simulink model "PubIfDecisionVSM_LngHMI"  (R2020b)
settings: Solver=FixedStepAuto  StartTime=0.0  StopTime=Inf  RelTol=1e-3
PostLoadFcn:
  | if any(exist('dsrtsu_mdlpostloadfcn', 'file') ~= 0), dsrtsu_mdlpostloadfcn('Execute', bdroot); end
InitFcn:
  | , if any(exist('dsmpb_private', 'file') ~= 0), dsmpb_private('dsmpb_mdlclblib', 'Init', bdroot); end,
PreSaveFcn:
  | , if any(exist('dsmpb_private', 'file') ~= 0), dsmpb_private('dsmpb_mdlclblib', 'PreSave', bdroot); end,
CloseFcn:
  | , if any(exist('dsmpb_private', 'file') ~= 0), dsmpb_private('dsmpb_mdlclblib', 'Close', bdroot); end,
settings Model: DataDictionary=HWA_DDs.sldd  RTICANMMDATA=struct('GeneralSetupData',struct('modelroot','F:\ADAS_Store\ADAS_Store\Adas\VSM\Long_HMI','generalsettings',struct('filesettings',struct('destfolder',struct('Name','RTICANMM_FILES','Check',1),'buildfolder',struct('Name','.','Check',1),'AbsDestfolder',struct('Name','F:\ADAS_Store\ADAS_Store\Adas\VSM\Long_HMI\RTICANMM_FILES'),'AbsBuildfolder',struct('Name','F:\ADAS_Store\ADAS_Store\Adas\VSM\Long_HMI'))),'options',struct('addpaths',1,'rmpaths',1,'addtrcexclusion',false,'cannavigator',struct('checkmonitoring',0),'show_usrtrc',0,'use_usrtrc',0),'advanced',struct('options',ones(1,100)),'MPSetup',{{}},'RTI',struct('Type','DSRT','Ver','4.2','Date','02-Nov-2019'),'modelname','PubIfDecisionVSM_LngHMI','block','PubIfDecisionVSM_LngHMI'))  DSRTSU_INTERNAL_RTIFPGA=150  Creator=GW00180895  LastModifiedBy=GW00199575
settings OptimizationCC: BlockReduction=off  ConditionallyExecuteInputs=off  OptimizeBlockIOStorage=off  BufferReuse=off  GlobalBufferReuse=off  ExpressionFolding=off  LocalBlockOutputs=off  OptimizeDataStoreBuffers=off  BusAssignmentInplaceUpdate=off
settings DebuggingCC: TasksWithSamePriorityMsg=none
settings HardwareCC: ProdBitPerPointer=32  ProdBitPerSizeT=32  ProdBitPerPtrDiffT=32  ProdLargestAtomicInteger=Integer  ProdWordSize=32  ProdHWDeviceType=Custom Processor->Custom
settings ModelReferenceCC: UpdateModelReferenceTargets=IfOutOfDate  EnableParallelModelReferenceBuilds=on  ModelReferenceNumInstancesAllowed=Single
settings SFSimCC: MATLABDynamicMemAlloc=off
settings RTWCC: Description=dSPACE Run-Time Target (for VEOS on Windows and ConfigurationDesk)  SystemTargetFile=dsrt.tlc  GenCodeOnly=on  MakeCommand=make_dsrt  TemplateMakefile=dsrt_default_tmf  RTWVerbose=off
settings CodeAppCC: MaxIdLength=128
settings STFCustomTargetCC: TargetLangStandard=C99 (ISO)  ParMdlRefBuildCompliant=on  ConcurrentExecutionCompliant=off  CPPClassGenCompliant=off  GRTInterface=off  SystemTargetFile=dsrt.tlc
settings GRTTargetCC: CompOptLevelCompliant=off  ConcurrentExecutionCompliant=off  CombineOutputUpdateFcns=off  MatFileLogging=off  CPPClassGenCompliant=off  UseToolchainInfoCompliant=off

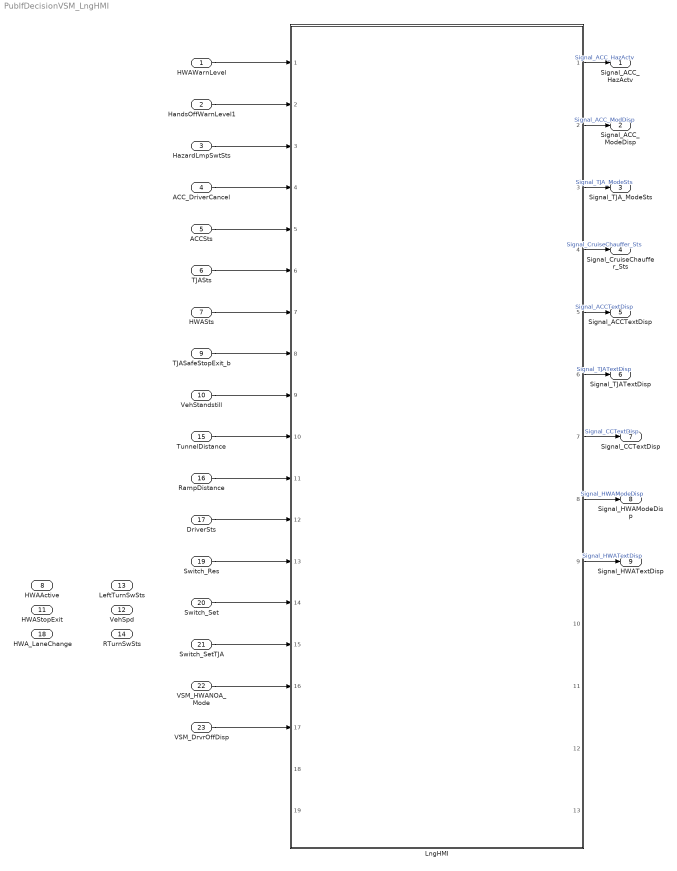
== system PubIfDecisionVSM_LngHMI ==
  HWAWarnLevel : Inport  OutDataTypeStr=uint8
  HandsOffWarnLevel1 : Inport  Port=2  OutDataTypeStr=uint8
  HazardLmpSwtSts : Inport  Port=3  OutDataTypeStr=boolean
  ACC_DriverCancel : Inport  Port=4  OutDataTypeStr=boolean
  ACCSts : Inport  Port=5  OutDataTypeStr=Enum: ACC_STATE
  TJASts : Inport  Port=6  OutDataTypeStr=Enum: TJA_STATE
  HWASts : Inport  Port=7  OutDataTypeStr=Enum: HWA_STATE
  HWAActive : Inport  Port=8  OutDataTypeStr=boolean
  TJASafeStopExit_b : Inport  Port=9  OutDataTypeStr=boolean
  VehStandstill : Inport  Port=10  OutDataTypeStr=uint8
  HWAStopExit : Inport  Port=11  OutDataTypeStr=boolean
  VehSpd : Inport  Port=12  OutDataTypeStr=single
  LeftTurnSwSts : Inport  Port=13  OutDataTypeStr=boolean
  RTurnSwSts : Inport  Port=14  OutDataTypeStr=boolean
  TunnelDistance : Inport  Port=15  OutDataTypeStr=uint16
  RampDistance : Inport  Port=16  OutDataTypeStr=uint16
  DriverSts : Inport  Port=17  OutDataTypeStr=uint8
  HWA_LaneChange : Inport  Port=18  OutDataTypeStr=uint8
  Switch_Res : Inport  Port=19  OutDataTypeStr=boolean
  Switch_Set : Inport  Port=20  OutDataTypeStr=boolean
  Switch_SetTJA : Inport  Port=21  OutDataTypeStr=boolean
  VSM_HWANOA_Mode : Inport  Port=22  OutDataTypeStr=boolean
  VSM_DrvrOffDisp : Inport  Port=23  OutDataTypeStr=boolean
  LngHMI : Subsystem  ReferencedSubsystem=PvtSubSys_VSM_LngHMI
  Signal_ACC_HazActv : Outport  OutDataTypeStr=uint8
  Signal_ACC_ModeDisp : Outport  Port=2  OutDataTypeStr=uint8
  Signal_TJA_ModeSts : Outport  Port=3  OutDataTypeStr=uint8
  Signal_CruiseChauffer_Sts : Outport  Port=4
  Signal_ACCTextDisp : Outport  Port=5  OutDataTypeStr=uint8
  Signal_TJATextDisp : Outport  Port=6  OutDataTypeStr=uint8
  Signal_CCTextDisp : Outport  Port=7
  Signal_HWAModeDisp : Outport  Port=8  OutDataTypeStr=uint8
  Signal_HWATextDisp : Outport  Port=9  OutDataTypeStr=uint8
  wires:
  LngHMI/9 -> Signal_HWATextDisp/1  "Signal_HWATextDisp"
  LngHMI/2 -> Signal_ACC_ModeDisp/1  "Signal_ACC_ModDisp"
  TJASts/1 -> LngHMI/6
  LngHMI/4 -> Signal_CruiseChauffer_Sts/1  "Signal_CruiseChauffer_Sts"
  LngHMI/7 -> Signal_CCTextDisp/1  "Signal_CCTextDisp"
  LngHMI/8 -> Signal_HWAModeDisp/1  "Signal_HWAModeDisp"
  LngHMI/5 -> Signal_ACCTextDisp/1  "Signal_ACCTextDisp"
  LngHMI/3 -> Signal_TJA_ModeSts/1  "Signal_TJA_ModeSts"
  ACCSts/1 -> LngHMI/5
  LngHMI/6 -> Signal_TJATextDisp/1  "Signal_TJATextDisp"
  LngHMI/1 -> Signal_ACC_HazActv/1  "Signal_ACC_HazActv"
  HWAWarnLevel/1 -> LngHMI/1
  ACC_DriverCancel/1 -> LngHMI/4
  HazardLmpSwtSts/1 -> LngHMI/3
  HandsOffWarnLevel1/1 -> LngHMI/2
  HWASts/1 -> LngHMI/7
  TJASafeStopExit_b/1 -> LngHMI/8
  VehStandstill/1 -> LngHMI/9
  TunnelDistance/1 -> LngHMI/10
  RampDistance/1 -> LngHMI/11
  DriverSts/1 -> LngHMI/12
  Switch_Res/1 -> LngHMI/13
  Switch_Set/1 -> LngHMI/14
  Switch_SetTJA/1 -> LngHMI/15
  VSM_HWANOA_Mode/1 -> LngHMI/16
  VSM_DrvrOffDisp/1 -> LngHMI/17
